simulink model "springmass"  (R2013a)
settings: Solver=ode45  StartTime=0.0  StopTime=10.0  MaxStep=.01  RelTol=1e-3
InitFcn:
  | springmass_params
values from neighbouring files (symbols this model uses):
  dy0 = -0.5    [springmass_params.m]
  k = 10000    [springmass_params.m]
  l0 = 1    [springmass_params.m]
  m = 70    [springmass_params.m]
  y0 = l0    (= 1)    [springmass_params.m]
libraries: simulink x1
settings Model: Creator=bshih1  LastModifiedBy=bshih1

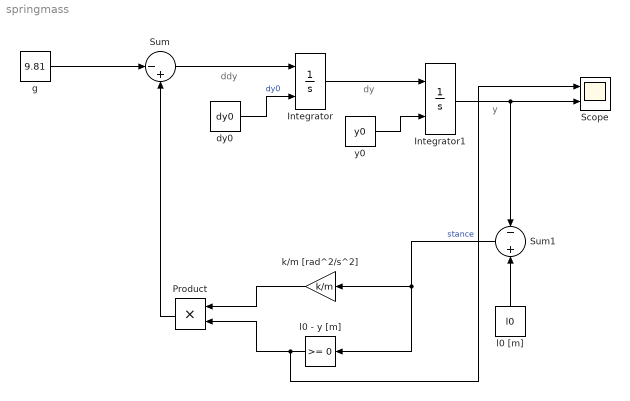
== system springmass ==
  note: ddy
  note: dy
  note: y
  Integrator : Integrator  InitialConditionSource=external
  Integrator1 : Integrator  InitialConditionSource=external
  Product : Product
  Scope : Scope  NumInputPorts=2
      settings: YMin=-5~-5  YMax=5~5
  Sum : Sum  Inputs=|-+
  Sum1 : Sum  Inputs=-+
  dy0 : Constant  Value=dy0
  g : Constant  Value=9.81
  k/m [rad^2/s^2] : Gain  Gain=k/m
  l0 - y [m] : simulink/Logic and Bit Operations/Compare To Zero  relop=>=  OutDataTypeStr=boolean
  l0 [m] : Constant  Value=l0
  y0 : Constant  Value=y0
  wires:
  g/1 -> Sum/1
  Integrator/1 -> Integrator1/1
  Sum/1 -> Integrator/1
  Product/1 -> Sum/2
  k/m [rad^2/s^2]/1 -> Product/1
  l0 - y [m]/1 -> Scope/1, Product/2  "stance"
  dy0/1 -> Integrator/2  "dy0"
  y0/1 -> Integrator1/2
  Sum1/1 -> l0 - y [m]/1, k/m [rad^2/s^2]/1
  Integrator1/1 -> Sum1/1, Scope/2
  l0 [m]/1 -> Sum1/2
